simulink model "hcu_main_ADASwEPS"  (Simulink 8.2)
settings: Solver=FixedStepDiscrete  StartTime=0.0  StopTime=inf  FixedStep=0.001  RelTol=1e-3
PostLoadFcn:
  | , if any(exist('dsrtsu_mdlpostloadfcn', 'file') == [2, 3, 6]), try dsrtsu_mdlpostloadfcn('Execute', bdroot); catch fprintf('Error in PostLoadFcn (dsrtsu_mdlpostloadfcn) for model "%s":\n %s\n', bdroot, lasterr); end, end,
values from neighbouring files (symbols this model uses):
  C_TASK_1MS_S = (	C_TICK_TIME_S       )    [hcu_local_hdr.m]    (also in temp_ovrd_values.m = double(	0.001                  ))
  C_TICK_TIME_S = single(	0.005	    	)    [hcu_local_hdr.m]
  ENUM_EPSLFCSTATUS_ACTIVE = uint8(  2  )    [hcu_local_hdr.m]
  ENUM_EPSLFCSTATUS_TRANSITION = uint8(  3  )    [hcu_local_hdr.m]
  ENUM_EPSLKASTATUS_ACTIVE = uint8(  2  )    [hcu_local_hdr.m]
  ENUM_EPSMODEREQ_ANGLE = uint8(  1  )    [hcu_local_hdr.m]
  ENUM_EPSMODEREQ_INTERNAL = uint8(  0  )    [hcu_local_hdr.m]
  ENUM_EPSMODEREQ_TORQUE = uint8(  2  )    [hcu_local_hdr.m]
  ENUM_GEARPOSN_1ST = uint8(  1  )    [hcu_local_hdr.m]
  ENUM_GEARPOSN_2ND = uint8(  2  )    [hcu_local_hdr.m]
  ENUM_GEARPOSN_3RD = uint8(  3  )    [hcu_local_hdr.m]
  ENUM_GEARPOSN_4TH = uint8(  4  )    [hcu_local_hdr.m]
  ENUM_GEARPOSN_5TH = uint8(  5  )    [hcu_local_hdr.m]
  ENUM_GEARPOSN_6TH = uint8(  6  )    [hcu_local_hdr.m]
  ENUM_GEARPOSN_R = uint8(  7  )    [hcu_local_hdr.m]
  FALSE = boolean( 0 )    [hcu_local_hdr.m]
  TRUE = boolean( 1 )    [hcu_local_hdr.m]
undefined symbols (not defined in the file or in its folder): AISP_EPSCurrent_pct, AISP_TqASensorDelta_pct, AISP_TqBSensorDelta_pct, dHAL_IN, hal, INVALID_ABS1_TIMEOUT, INVALID_ABS2_TIMEOUT, INVALID_ABS3_TIMEOUT, INVALID_ABS4_TIMEOUT, INVALID_AC1_TIMEOUT, INVALID_ADASTORQ_REQ, INVALID_BCM1_TIMEOUT, INVALID_BCM2_TIMEOUT, INVALID_BOOSTER_VAC, INVALID_CSW1_TIMEOUT, INVALID_CUR_VEHDECE, INVALID_CURBRAKEDECE_REQ, INVALID_CURSTEERANG_REQ, INVALID_CURSTEERTQ_REQ, INVALID_ECM1_TIMEOUT, INVALID_ECM2_TIMEOUT, INVALID_ECM3_TIMEOUT, INVALID_ECM9_TIMEOUT, INVALID_ENG_TORQUE_FRICTIONAL, INVALID_ENG_TORQUE_INDICATED, INVALID_ENG_TORQUE_INDICATEDCOR, INVALID_ENG_TQ_MAX, INVALID_ENG_TQ_MIN, INVALID_EPAS2_TIMEOUT, INVALID_EPAS3_TIMEOUT, INVALID_EPB1_TIMEOUT, INVALID_EPS_BATTVOLT, INVALID_ESC_BATTVOLT, INVALID_GRADE, INVALID_HCU3_TIMEOUT, INVALID_HCU4_TIMEOUT, INVALID_HMI1_TIMEOUT, INVALID_HMI2_TIMEOUT, INVALID_LAT_ACC, INVALID_LONG_ACC, INVALID_MC_PRESSURE, INVALID_METER1_TIMEOUT, INVALID_METER3_TIMEOUT, INVALID_METER_VEHSPD, INVALID_ODO_METER, INVALID_OUTSIDE_TEMP, INVALID_PARKBRAKEBIND_STAT, INVALID_PEDALTQ_REQ, INVALID_SAS1_TIMEOUT, INVALID_SAS_ANGLE, INVALID_SHIFTER_POSN, INVALID_TCM1_TIMEOUT, INVALID_TCM2_TIMEOUT, INVALID_VCU1_TIMEOUT, INVALID_VCU2_TIMEOUT, INVALID_VEH_CRASH, INVALID_VEH_SPD, INVALID_WHEEL_SPD, INVALID_YAW_RATE, KHAL_MssgIdObj1_num ... (+8)
libraries: simulink x147, hcu_lib x38, rti1401lib_dio_type3 x4, rtimmsu_dsrtlib x3, app x1, rtiethernetudplib x1, rti1401lib_adc_type4 x1, rti1401lib_dac_type3 x1, inp x1, lidr x1, outp x1
(part 13 of 15)

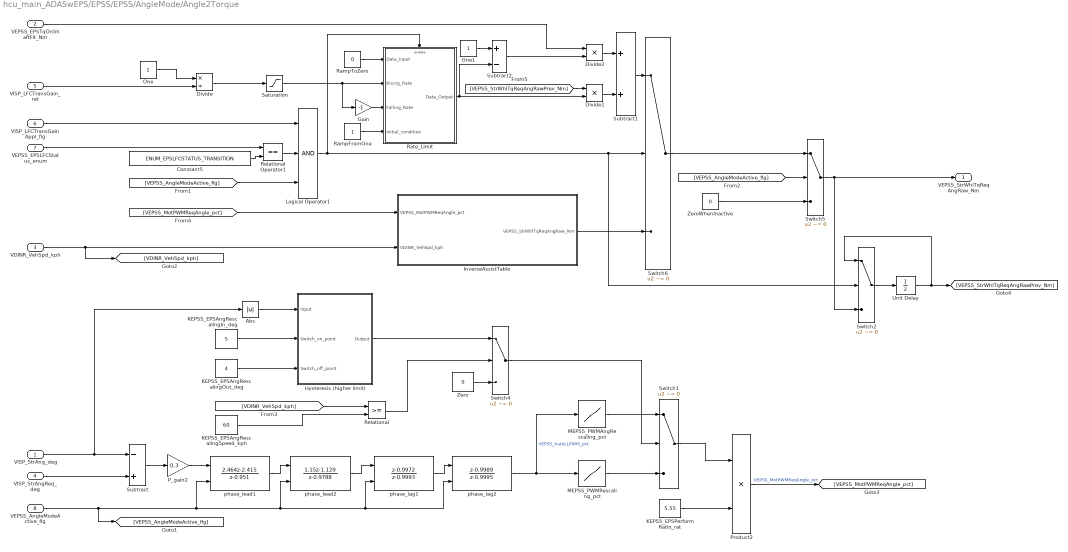
== system hcu_main_ADASwEPS/EPSS/EPSS/AngleMode/Angle2Torque ==
  VISP_StrAng_deg : Inport
  VEPSS_EPSTqOnShaftFlt_Nm : Inport  Port=2
  VDINR_VehSpd_kph : Inport  Port=3
  VISP_StrAngReq_deg : Inport  Port=4
  VISP_LFCTransGain_rat : Inport  Port=5
  VISP_LFCTransGainAppl_flg : Inport  Port=6
  VEPSS_EPSLFCStatus_enum : Inport  Port=7
  VEPSS_AngleModeActive_flg : Inport  Port=8
  Abs : Abs
  Constant5 : Constant  Value=ENUM_EPSLFCSTATUS_TRANSITION
  Divide : Product  Inputs=*/
  Divide1 : Product  Inputs=**
  Divide2 : Product  Inputs=**
  Gain : Gain  Gain=-1
  Hysteresis (higher limit) : Subsystem  TreatAsAtomicUnit=on
  InverseAssistTable : Subsystem
  KEPSS_EPSAngRescalingIn_deg : Constant  Value=5  SampleTime=-1
  KEPSS_EPSAngRescalingOut_deg : Constant  Value=4  SampleTime=-1
  KEPSS_EPSAngRescalingSpeed_kph : Constant  Value=60  SampleTime=-1
  KEPSS_EPSPerformRatio_rat : Constant  Value=5.55  SampleTime=-1
  Logical Operator1 : Logic  Inputs=3  AllPortsSameDT=off  OutDataTypeStr=boolean
  MEPSS_PWMAngRescaling_pct : Lookup  InputValues=[-100 -0.1 0 0.1 100]  Table=[-100 -0.1 0 0.1 100]  LookUpMeth=Interpolation-Use End Values
      settings: AttributesFormatString="Input=\"%<InputValues>\"\\nOutput=\"%<Table>\""
  MEPSS_PWMRescaling_pct : Lookup  InputValues=[-100 -0.1 0 0.1 100]  Table=[-100 -2.2 0 2.6 100]  LookUpMeth=Interpolation-Use End Values
      settings: AttributesFormatString="Input=\"%<InputValues>\"\\nOutput=\"%<Table>\""
  One : Constant
  One1 : Constant
  P_gain2 : Gain  Gain=0.3
  Product2 : Product  RndMeth=Zero
  RampFromOne : Constant
  RampToZero : Constant  Value=0
  Rate_Limit : Subsystem  TreatAsAtomicUnit=on
  "Relational " : RelationalOperator  OutDataTypeStr=boolean
  Relational Operator1 : RelationalOperator  Operator===  OutDataTypeStr=boolean
  Saturation : Saturate  UpperLimit=inf  LowerLimit=0
  Subtract : Sum  Inputs=-+
  Subtract1 : Sum
  Subtract2 : Sum  Inputs=+-
  Switch{1..2,4..6} (5 alike) : Switch  Criteria=u2 ~= 0
  Unit Delay : UnitDelay  SampleTime=-1
  Zero : Constant  Value=0  SampleTime=-1
  ZeroWhenInactive : Constant  Value=0
  phase_lag1 : DiscreteTransferFcn  Numerator=[1 -0.9972]  Denominator=[1 -0.9993]  ExternalReset=Rising
      settings: InputPortMap=u0,r7
  phase_lag2 : DiscreteTransferFcn  Numerator=[1 -0.9989]  Denominator=[1 -0.9995]  ExternalReset=Rising
      settings: InputPortMap=u0,r7
  phase_lead1 : DiscreteTransferFcn  Numerator=[2.464 -2.415]  Denominator=[1 -0.951]  ExternalReset=Rising
      settings: InputPortMap=u0,r7
  phase_lead2 : DiscreteTransferFcn  Numerator=[1.15 -1.129]  Denominator=[1 -0.9788]  ExternalReset=Rising
      settings: InputPortMap=u0,r7
  VEPSS_StrWhlTqReqAngRaw_Nm : Outport
  wires:
  phase_lag2/1 -> MEPSS_PWMRescaling_pct/1, MEPSS_PWMAngRescaling_pct/1  "VEPSS_AutoLLPWM_pct"
  VISP_StrAng_deg/1 -> Subtract/1, Abs/1
  KEPSS_EPSPerformRatio_rat/1 -> Product2/2
  VISP_StrAngReq_deg/1 -> Subtract/2
  MEPSS_PWMRescaling_pct/1 -> Switch1/3
  Product2/1 -> [VEPSS_MotPWMReqAngle_pct]  "VEPSS_MotPWMReqAngle_pct"
  Subtract/1 -> P_gain2/1
  P_gain2/1 -> phase_lead1/1
  phase_lead1/1 -> phase_lead2/1
  phase_lag1/1 -> phase_lag2/1
  phase_lead2/1 -> phase_lag1/1
  MEPSS_PWMAngRescaling_pct/1 -> Switch1/1
  Switch1/1 -> Product2/1
  Switch4/1 -> Switch1/2
  KEPSS_EPSAngRescalingSpeed_kph/1 -> "Relational "/2
  "Relational "/1 -> Switch4/2
  Zero/1 -> Switch4/3
  VEPSS_EPSLFCStatus_enum/1 -> Relational Operator1/1
  Constant5/1 -> Relational Operator1/2
  VISP_LFCTransGainAppl_flg/1 -> Logical Operator1/1
  Relational Operator1/1 -> Logical Operator1/2
  VEPSS_AngleModeActive_flg/1 -> phase_lead2/2, phase_lag2/2, phase_lag1/2, phase_lead1/2, [VEPSS_AngleModeActive_flg]
  InverseAssistTable/1(VEPSS_StrWhlTqReqAngRaw_Nm) -> Switch6/3
  RampToZero/1 -> Rate_Limit/1(Data_Input)
  RampFromOne/1 -> Rate_Limit/4(Initial_condition)
  Logical Operator1/1 -> Switch2/2, Switch6/2, Rate_Limit/Enable
  Divide/1 -> Saturation/1
  Gain/1 -> Rate_Limit/3(Falling_Rate)
  [VEPSS_AngleModeActive_flg] -> Logical Operator1/3
  Switch6/1 -> Switch5/1
  Switch5/1 -> Switch2/3, VEPSS_StrWhlTqReqAngRaw_Nm/1
  [VEPSS_AngleModeActive_flg] -> Switch5/2
  ZeroWhenInactive/1 -> Switch5/3
  VDINR_VehSpd_kph/1 -> [VDINR_VehSpd_kph], InverseAssistTable/2(VDINR_VehSpd_kph)
  [VDINR_VehSpd_kph] -> "Relational "/1
  Abs/1 -> Hysteresis (higher limit)/1(Input)
  KEPSS_EPSAngRescalingIn_deg/1 -> Hysteresis (higher limit)/2(Switch_on_point)
  KEPSS_EPSAngRescalingOut_deg/1 -> Hysteresis (higher limit)/3(Switch_off_point)
  Hysteresis (higher limit)/1(Output) -> Switch4/1
  [VEPSS_MotPWMReqAngle_pct] -> InverseAssistTable/1(VEPSS_MotPWMReqAngle_pct)
  VEPSS_EPSTqOnShaftFlt_Nm/1 -> Divide2/1
  VISP_LFCTransGain_rat/1 -> Divide/2
  One/1 -> Divide/1
  Saturation/1 -> Gain/1, Rate_Limit/2(Rising_Rate)
  Subtract1/1 -> Switch6/1
  Divide1/1 -> Subtract1/2
  Rate_Limit/1(Data_Output) -> Subtract2/2, Divide1/2
  Divide2/1 -> Subtract1/1
  [VEPSS_StrWhlTqReqAngRawPrev_Nm] -> Divide1/1
  Subtract2/1 -> Divide2/2
  One1/1 -> Subtract2/1
  Switch2/1 -> Unit Delay/1
  Unit Delay/1 -> Switch2/1, [VEPSS_StrWhlTqReqAngRawPrev_Nm]

== system hcu_main_ADASwEPS/EPSS/EPSS/EPSMotorPWMRequest/MotorPWMRequestCalculation ==
  VEPSS_EPSMotTqReqRaw_Nm : Inport
  1/KEPSS_PWM2TqGain_rat : Gain
  VEPSS_EPSMotPWMReqRaw_pct : Outport
  wires:
  1/KEPSS_PWM2TqGain_rat/1 -> VEPSS_EPSMotPWMReqRaw_pct/1  "VEPSS_EPSMotPWMReqRaw_pct"
  VEPSS_EPSMotTqReqRaw_Nm/1 -> 1/KEPSS_PWM2TqGain_rat/1

== system hcu_main_ADASwEPS/EPSS/EPSS/EPSMotorPWMRequest/MotorTorqueRequestCalculation ==
  VEPSS_StrWhlTqReqAst_Nm : Inport
  VEPSS_StrWhlTqReqTq_Nm : Inport  Port=2
  VEPSS_StrWhlTqReqAng_Nm : Inport  Port=3
  VEPSS_TorqueModeActive_flg : Inport  Port=4
  VEPSS_AngleModeActive_flg : Inport  Port=5
  VISP_VehSpd_kph : Inport  Port=6
  VISP_LFCTransGain_rat : Inport  Port=7
  VISP_LFCTransGainAppl_flg : Inport  Port=8
  VEPSS_EPSLFCStatus_enum : Inport  Port=9
  VISP_EPSModeReq_enum : Inport  Port=10
  EPSGainDefault : Constant
  KEPSS_PWM2TqGain_rat : Gain
  MEPSS_MotorPWMRescaling_pct : Lookup  InputValues=[-100 -3 0 3 100]  Table=[-250 -3 0 3 250]  LookUpMeth=Interpolation-Use End Values
      settings: AttributesFormatString="Input=\"%<InputValues>\"\\nOutput=\"%<Table>\""
  MEPSS_TqPWMMult_rat : Lookup  InputValues=[-100 -80 -60 -40 -20 -10 0 10 20 40 60 80 100]  Table=[1 1 1 1 1 1 1 1 1 1 1 1 1]  LookUpMeth=Interpolation-Use End Values
      settings: AttributesFormatString="Input=\"%<InputValues>\"\\nOutput=\"%<Table>\""
  MEPSS_TqPWM_pct : Lookup  InputValues=[-10:0.5:10]  Table="[-100\t-95\t-90\t-85\t-80\t-75\t-70\t-65\t-60\t-55\t-50\t-45\t-40\t-35\t-30\t-25\t-20\t-15\t-10\t-5\t0\t5\t10\t15\t20\t25\t30\t35\t40\t45\t50\t55\t60\t65\t70\t75\t80\t85\t90\t95\t100]"  LookUpMeth=Interpolation-Use End Values
      settings: AttributesFormatString="Input=\"%<InputValues>\"\\nOutput=\"%<Table>\""
  Product1 : Product  Inputs=3
  Switch : Switch  Criteria=u2 ~= 0
  Switch1 : Switch  Criteria=u2 ~= 0
  Terminator{,1..3} (4 alike) : Terminator
  VEPSS_EPSMotTqReq_Nm : Outport
  wires:
  MEPSS_TqPWMMult_rat/1 -> Product1/2
  MEPSS_TqPWM_pct/1 -> Product1/1
  VISP_VehSpd_kph/1 -> MEPSS_TqPWMMult_rat/1
  Product1/1 -> MEPSS_MotorPWMRescaling_pct/1
  VEPSS_AngleModeActive_flg/1 -> Switch/2
  VEPSS_StrWhlTqReqAng_Nm/1 -> Switch/1
  Switch1/1 -> Switch/3
  VEPSS_TorqueModeActive_flg/1 -> Switch1/2
  VEPSS_StrWhlTqReqTq_Nm/1 -> Switch1/1
  VEPSS_StrWhlTqReqAst_Nm/1 -> Switch1/3
  Switch/1 -> MEPSS_TqPWM_pct/1
  EPSGainDefault/1 -> Product1/3  "VEPSS_MotTqGain_rat"
  MEPSS_MotorPWMRescaling_pct/1 -> KEPSS_PWM2TqGain_rat/1
  KEPSS_PWM2TqGain_rat/1 -> VEPSS_EPSMotTqReq_Nm/1  "VEPSS_EPSMotTqReq_Nm"
  VISP_LFCTransGain_rat/1 -> Terminator/1
  VISP_LFCTransGainAppl_flg/1 -> Terminator1/1
  VEPSS_EPSLFCStatus_enum/1 -> Terminator2/1
  VISP_EPSModeReq_enum/1 -> Terminator3/1

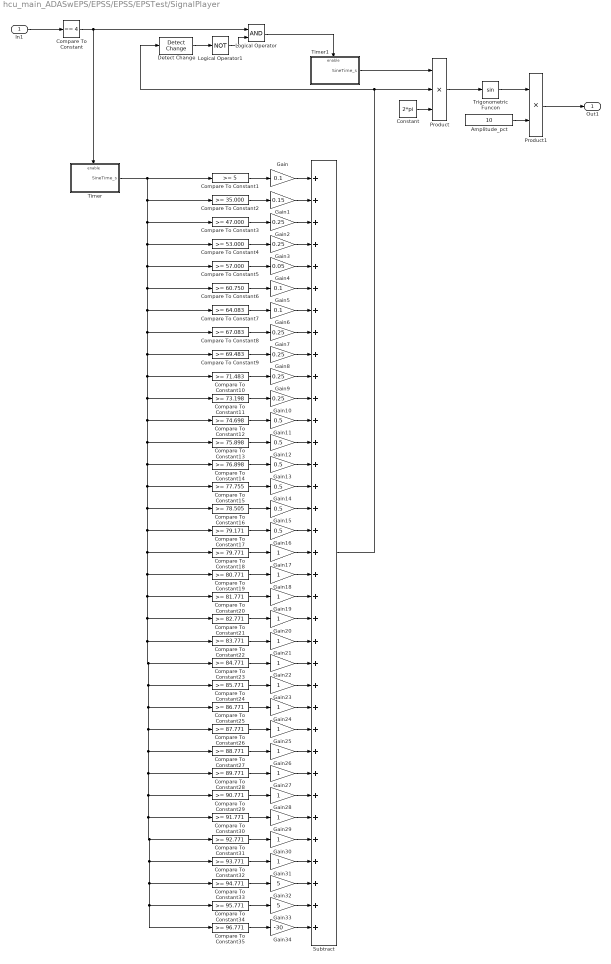
== system hcu_main_ADASwEPS/EPSS/EPSS/EPSTest/SignalPlayer ==
  In1 : Inport
  Amplitude_pct : Constant  Value=10
  Compare To Constant : simulink/Logic and Bit Operations/Compare To Constant  relop===  const=4  OutDataTypeStr=boolean
  Compare To Constant1 : simulink/Logic and Bit Operations/Compare To Constant  relop=>=  const=5  OutDataTypeStr=boolean
  Compare To Constant10 : simulink/Logic and Bit Operations/Compare To Constant  relop=>=  const=71.483  OutDataTypeStr=boolean
  Compare To Constant11 : simulink/Logic and Bit Operations/Compare To Constant  relop=>=  const=73.198  OutDataTypeStr=boolean
  Compare To Constant12 : simulink/Logic and Bit Operations/Compare To Constant  relop=>=  const=74.698  OutDataTypeStr=boolean
  Compare To Constant13 : simulink/Logic and Bit Operations/Compare To Constant  relop=>=  const=75.898  OutDataTypeStr=boolean
  Compare To Constant14 : simulink/Logic and Bit Operations/Compare To Constant  relop=>=  const=76.898  OutDataTypeStr=boolean
  Compare To Constant15 : simulink/Logic and Bit Operations/Compare To Constant  relop=>=  const=77.755  OutDataTypeStr=boolean
  Compare To Constant16 : simulink/Logic and Bit Operations/Compare To Constant  relop=>=  const=78.505  OutDataTypeStr=boolean
  Compare To Constant17 : simulink/Logic and Bit Operations/Compare To Constant  relop=>=  const=79.171  OutDataTypeStr=boolean
  Compare To Constant18 : simulink/Logic and Bit Operations/Compare To Constant  relop=>=  const=79.771  OutDataTypeStr=boolean
  Compare To Constant19 : simulink/Logic and Bit Operations/Compare To Constant  relop=>=  const=80.771  OutDataTypeStr=boolean
  Compare To Constant2 : simulink/Logic and Bit Operations/Compare To Constant  relop=>=  const=35.000  OutDataTypeStr=boolean
  Compare To Constant20 : simulink/Logic and Bit Operations/Compare To Constant  relop=>=  const=81.771  OutDataTypeStr=boolean
  Compare To Constant21 : simulink/Logic and Bit Operations/Compare To Constant  relop=>=  const=82.771  OutDataTypeStr=boolean
  Compare To Constant22 : simulink/Logic and Bit Operations/Compare To Constant  relop=>=  const=83.771  OutDataTypeStr=boolean
  Compare To Constant23 : simulink/Logic and Bit Operations/Compare To Constant  relop=>=  const=84.771  OutDataTypeStr=boolean
  Compare To Constant24 : simulink/Logic and Bit Operations/Compare To Constant  relop=>=  const=85.771  OutDataTypeStr=boolean
  Compare To Constant25 : simulink/Logic and Bit Operations/Compare To Constant  relop=>=  const=86.771  OutDataTypeStr=boolean
  Compare To Constant26 : simulink/Logic and Bit Operations/Compare To Constant  relop=>=  const=87.771  OutDataTypeStr=boolean
  Compare To Constant27 : simulink/Logic and Bit Operations/Compare To Constant  relop=>=  const=88.771  OutDataTypeStr=boolean
  Compare To Constant28 : simulink/Logic and Bit Operations/Compare To Constant  relop=>=  const=89.771  OutDataTypeStr=boolean
  Compare To Constant29 : simulink/Logic and Bit Operations/Compare To Constant  relop=>=  const=90.771  OutDataTypeStr=boolean
  Compare To Constant3 : simulink/Logic and Bit Operations/Compare To Constant  relop=>=  const=47.000  OutDataTypeStr=boolean
  Compare To Constant30 : simulink/Logic and Bit Operations/Compare To Constant  relop=>=  const=91.771  OutDataTypeStr=boolean
  Compare To Constant31 : simulink/Logic and Bit Operations/Compare To Constant  relop=>=  const=92.771  OutDataTypeStr=boolean
  Compare To Constant32 : simulink/Logic and Bit Operations/Compare To Constant  relop=>=  const=93.771  OutDataTypeStr=boolean
  Compare To Constant33 : simulink/Logic and Bit Operations/Compare To Constant  relop=>=  const=94.771  OutDataTypeStr=boolean
  Compare To Constant34 : simulink/Logic and Bit Operations/Compare To Constant  relop=>=  const=95.771  OutDataTypeStr=boolean
  Compare To Constant35 : simulink/Logic and Bit Operations/Compare To Constant  relop=>=  const=96.771  OutDataTypeStr=boolean
  Compare To Constant4 : simulink/Logic and Bit Operations/Compare To Constant  relop=>=  const=53.000  OutDataTypeStr=boolean
  Compare To Constant5 : simulink/Logic and Bit Operations/Compare To Constant  relop=>=  const=57.000  OutDataTypeStr=boolean
  Compare To Constant6 : simulink/Logic and Bit Operations/Compare To Constant  relop=>=  const=60.750  OutDataTypeStr=boolean
  Compare To Constant7 : simulink/Logic and Bit Operations/Compare To Constant  relop=>=  const=64.083  OutDataTypeStr=boolean
  Compare To Constant8 : simulink/Logic and Bit Operations/Compare To Constant  relop=>=  const=67.083  OutDataTypeStr=boolean
  Compare To Constant9 : simulink/Logic and Bit Operations/Compare To Constant  relop=>=  const=69.483  OutDataTypeStr=boolean
  Constant : Constant  Value=2*pi  OutDataTypeStr=single
  Detect Change : simulink/Logic and Bit Operations/Detect Change  vinit=0  InputProcessing=Inherited  OutDataTypeStr=boolean
  Gain : Gain  Gain=0.1
  Gain1 : Gain  Gain=0.15
  Gain{2..3,7..10} (6 alike) : Gain  Gain=0.25
  Gain{11..16} (6 alike) : Gain  Gain=0.5
  Gain{17..31} (15 alike) : Gain
  Gain32 : Gain  Gain=5
  Gain33 : Gain  Gain=5
  Gain34 : Gain  Gain=-30
  Gain4 : Gain  Gain=0.05
  Gain5 : Gain  Gain=0.1
  Gain6 : Gain  Gain=0.1
  Logical Operator : Logic  AllPortsSameDT=off  OutDataTypeStr=boolean
  Logical Operator1 : Logic  Operator=NOT  AllPortsSameDT=off  OutDataTypeStr=boolean
  Product : Product  Inputs=3  RndMeth=Zero
  Product1 : Product  RndMeth=Zero
  Subtract : Sum  Inputs=35
  Timer : Subsystem
  Timer1 : Subsystem
  Trigonometric Funcon : Trigonometry
  Out1 : Outport
  wires:
  Subtract/1 -> Product/2, Detect Change/1
  Product/1 -> Trigonometric Funcon/1
  Amplitude_pct/1 -> Product1/2
  Trigonometric Funcon/1 -> Product1/1
  Constant/1 -> Product/3
  Compare To Constant/1 -> Logical Operator/1, Timer/Enable
  In1/1 -> Compare To Constant/1
  Timer/1(SineTime_s) -> Compare To Constant2/1, Compare To Constant8/1, Compare To Constant35/1, Compare To Constant34/1, Compare To Constant33/1, Compare To Constant32/1, Compare To Constant31/1, Compare To Constant30/1, Compare To Constant29/1, Compare To Constant28/1, Compare To Constant27/1, Compare To Constant26/1, Compare To Constant25/1, Compare To Constant24/1, Compare To Constant23/1, Compare To Constant22/1, Compare To Constant21/1, Compare To Constant20/1, Compare To Constant19/1, Compare To Constant18/1, Compare To Constant17/1, Compare To Constant16/1, Compare To Constant15/1, Compare To Constant14/1, Compare To Constant13/1, Compare To Constant12/1, Compare To Constant11/1, Compare To Constant10/1, Compare To Constant9/1, Compare To Constant7/1, Compare To Constant6/1, Compare To Constant5/1, Compare To Constant4/1, Compare To Constant3/1, Compare To Constant1/1
  Compare To Constant1/1 -> Gain/1
  Gain/1 -> Subtract/1
  Compare To Constant2/1 -> Gain1/1
  Gain1/1 -> Subtract/2
  Compare To Constant3/1 -> Gain2/1
  Gain2/1 -> Subtract/3
  Compare To Constant4/1 -> Gain3/1
  Gain3/1 -> Subtract/4
  Compare To Constant5/1 -> Gain4/1
  Gain4/1 -> Subtract/5
  Compare To Constant6/1 -> Gain5/1
  Gain5/1 -> Subtract/6
  Compare To Constant7/1 -> Gain6/1
  Gain6/1 -> Subtract/7
  Compare To Constant8/1 -> Gain7/1
  Gain7/1 -> Subtract/8
  Compare To Constant9/1 -> Gain8/1
  Gain8/1 -> Subtract/9
  Compare To Constant10/1 -> Gain9/1
  Gain9/1 -> Subtract/10
  Compare To Constant11/1 -> Gain10/1
  Gain10/1 -> Subtract/11
  Compare To Constant12/1 -> Gain11/1
  Gain11/1 -> Subtract/12
  Compare To Constant13/1 -> Gain12/1
  Gain12/1 -> Subtract/13
  Compare To Constant14/1 -> Gain13/1
  Gain13/1 -> Subtract/14
  Compare To Constant15/1 -> Gain14/1
  Gain14/1 -> Subtract/15
  Compare To Constant16/1 -> Gain15/1
  Gain15/1 -> Subtract/16
  Compare To Constant17/1 -> Gain16/1
  Gain16/1 -> Subtract/17
  Compare To Constant18/1 -> Gain17/1
  Gain17/1 -> Subtract/18
  Compare To Constant19/1 -> Gain18/1
  Gain18/1 -> Subtract/19
  Compare To Constant20/1 -> Gain19/1
  Gain19/1 -> Subtract/20
  Compare To Constant21/1 -> Gain20/1
  Gain20/1 -> Subtract/21
  Compare To Constant22/1 -> Gain21/1
  Gain21/1 -> Subtract/22
  Compare To Constant23/1 -> Gain22/1
  Gain22/1 -> Subtract/23
  Compare To Constant24/1 -> Gain23/1
  Gain23/1 -> Subtract/24
  Compare To Constant25/1 -> Gain24/1
  Gain24/1 -> Subtract/25
  Compare To Constant26/1 -> Gain25/1
  Gain25/1 -> Subtract/26
  Compare To Constant27/1 -> Gain26/1
  Gain26/1 -> Subtract/27
  Compare To Constant28/1 -> Gain27/1
  Gain27/1 -> Subtract/28
  Compare To Constant29/1 -> Gain28/1
  Gain28/1 -> Subtract/29
  Compare To Constant30/1 -> Gain29/1
  Gain29/1 -> Subtract/30
  Compare To Constant31/1 -> Gain30/1
  Gain30/1 -> Subtract/31
  Compare To Constant32/1 -> Gain31/1
  Gain31/1 -> Subtract/32
  Compare To Constant33/1 -> Gain32/1
  Gain32/1 -> Subtract/33
  Compare To Constant34/1 -> Gain33/1
  Gain33/1 -> Subtract/34
  Compare To Constant35/1 -> Gain34/1
  Gain34/1 -> Subtract/35
  Product1/1 -> Out1/1
  Timer1/1(SineTime_s) -> Product/1
  Logical Operator/1 -> Timer1/Enable
  Detect Change/1 -> Logical Operator1/1
  Logical Operator1/1 -> Logical Operator/2

== system hcu_main_ADASwEPS/EPSS/EPSS/EPSTest/Timer ==
  Enable : EnablePort  StatesWhenEnabling=reset
  C_TASK_1MS_S : Constant  Value=C_TASK_1MS_S
  Sum : Sum  Inputs=|++
  Unit Delay : UnitDelay  SampleTime=-1
  Unit Delay1 : UnitDelay  SampleTime=-1
  SineTime_s : Outport  OutputWhenDisabled=reset  InitialOutput=[0]
  wires:
  Unit Delay1/1 -> Sum/1
  Unit Delay/1 -> Sum/2
  Sum/1 -> SineTime_s/1, Unit Delay/1  "SineTime_s"
  C_TASK_1MS_S/1 -> Unit Delay1/1

== system hcu_main_ADASwEPS/ISP/PassThrough/EPSDegTest/Timer ==
  Enable : EnablePort  StatesWhenEnabling=reset
  C_TASK_1MS_S : Constant  Value=C_TASK_1MS_S
  Sum : Sum  Inputs=|++
  Unit Delay : UnitDelay  SampleTime=-1
  Unit Delay1 : UnitDelay  SampleTime=-1
  SineTime_s : Outport  OutputWhenDisabled=reset  InitialOutput=[0]
  wires:
  Unit Delay1/1 -> Sum/1
  Unit Delay/1 -> Sum/2
  Sum/1 -> SineTime_s/1, Unit Delay/1  "SineTime_s"
  C_TASK_1MS_S/1 -> Unit Delay1/1

== system hcu_main_ADASwEPS/ISP/TqProcessing/TqSensorAZero/Latch ==
  in : Inport
  update : Inport  Port=2
  Delay : Delay  DelayLength=1  InitialCondition=50
  Switch2 : Switch  Criteria=u2 ~= 0  Threshold=0.5
      settings: AttributesFormatString=<Criteria=%<Criteria>>
  out : Outport
  wires:
  Delay/1 -> Switch2/3
  in/1 -> Switch2/1
  Switch2/1 -> out/1, Delay/1
  update/1 -> Switch2/2

== system hcu_main_ADASwEPS/ISP/TqProcessing/TqSensorAZero/Timer ==
  Enable : EnablePort  StatesWhenEnabling=reset
  C_TASK_1MS_S : Constant  Value=C_TASK_1MS_S
  Sum : Sum  Inputs=|++
  Unit Delay : UnitDelay  SampleTime=-1
  Unit Delay1 : UnitDelay  SampleTime=-1
  Time_s : Outport  OutputWhenDisabled=reset  InitialOutput=[0]
  wires:
  Unit Delay1/1 -> Sum/1
  Unit Delay/1 -> Sum/2
  Sum/1 -> Time_s/1, Unit Delay/1  "Time_s"
  C_TASK_1MS_S/1 -> Unit Delay1/1

== system hcu_main_ADASwEPS/ISP/TqProcessing/TqSensorBZero/Latch ==
  in : Inport
  update : Inport  Port=2
  Delay : Delay  DelayLength=1  InitialCondition=50
  Switch2 : Switch  Criteria=u2 ~= 0  Threshold=0.5
      settings: AttributesFormatString=<Criteria=%<Criteria>>
  out : Outport
  wires:
  update/1 -> Switch2/2
  Switch2/1 -> Delay/1, out/1
  in/1 -> Switch2/1
  Delay/1 -> Switch2/3

== system hcu_main_ADASwEPS/ISP/TqProcessing/TqSensorBZero/Timer ==
  Enable : EnablePort  StatesWhenEnabling=reset
  C_TASK_1MS_S : Constant  Value=C_TASK_1MS_S
  Sum : Sum  Inputs=|++
  Unit Delay : UnitDelay  SampleTime=-1
  Unit Delay1 : UnitDelay  SampleTime=-1
  Time_s : Outport  OutputWhenDisabled=reset  InitialOutput=[0]
  wires:
  C_TASK_1MS_S/1 -> Unit Delay1/1
  Sum/1 -> Unit Delay/1, Time_s/1  "Time_s"
  Unit Delay/1 -> Sum/2
  Unit Delay1/1 -> Sum/1

== system hcu_main_ADASwEPS/OSP/OSP/CheckSum Calculation/Byte0 ==
  BISP_outputs : Inport
  Bus Selector : BusSelector  OutputSignals=VISP_StrAng_deg
  Data Type Conversion : DataTypeConversion  OutDataTypeStr=uint16
  Data Type Conversion1 : DataTypeConversion  OutDataTypeStr=uint16
  Data Type Conversion2 : DataTypeConversion  OutDataTypeStr=uint8
  Data Type Conversion3 : DataTypeConversion  OutDataTypeStr=uint8
  Extract Bits : simulink/Logic and Bit Operations/Extract Bits  bitsToExtract=Upper half  numBits=8  bitIdxRange=[0 7]  outScalingMode=Preserve fixed-point scaling
  Extract Bits1 : simulink/Logic and Bit Operations/Extract Bits  bitsToExtract=Lower half  numBits=8  bitIdxRange=[0 7]  outScalingMode=Preserve fixed-point scaling
  SAS_Angle_cvt : Subsystem  mask(ConvertOut){gain=0.1, offset=-900}
      mask help:
      | Conversion Formula
      |
      | The conversion formula is
      |
      | raw_value = (physical_value - Offset) / Factor
      |
      | where physical_value is the value of the signal after it is saturated using the specified Min and Max values. raw_value is the packed signal value.
  Shift Arithmetic : ArithShift  BitShiftNumber=8
  Byte0 : Outport
  ForByte1 : Outport  Port=2
  wires:
  BISP_outputs/1 -> Bus Selector/1
  Bus Selector/1 -> SAS_Angle_cvt/1(value)  "<VISP_StrAng_deg>"
  SAS_Angle_cvt/1(raw32) -> Data Type Conversion/1
  Data Type Conversion2/1 -> ForByte1/1
  Data Type Conversion1/1 -> Shift Arithmetic/1
  Extract Bits/1 -> Data Type Conversion1/1
  Shift Arithmetic/1 -> Data Type Conversion3/1
  Data Type Conversion3/1 -> Byte0/1
  Extract Bits1/1 -> Data Type Conversion2/1
  Data Type Conversion/1 -> Extract Bits/1, Extract Bits1/1

== system hcu_main_ADASwEPS/OSP/OSP/CheckSum Calculation/Byte1 ==
  ForByte1 : Inport
  Data Type Conversion3 : DataTypeConversion  OutDataTypeStr=uint8
  Byte1 : Outport
  wires:
  Data Type Conversion3/1 -> Byte1/1
  ForByte1/1 -> Data Type Conversion3/1

== system hcu_main_ADASwEPS/OSP/OSP/CheckSum Calculation/Byte2 ==
  Constant1 : Constant  Value=0
  Data Type Conversion3 : DataTypeConversion  OutDataTypeStr=uint8
  Byte2 : Outport
  wires:
  Constant1/1 -> Data Type Conversion3/1
  Data Type Conversion3/1 -> Byte2/1

== system hcu_main_ADASwEPS/OSP/OSP/CheckSum Calculation/Byte3 ==
  BISP_outputs : Inport
  Bus Selector : BusSelector  OutputSignals=VISP_StrAngSensorValid_flg,VISP_StrAngValid_flg
  Data Type Conversion1 : DataTypeConversion  OutDataTypeStr=uint8
  Data Type Conversion2 : DataTypeConversion  OutDataTypeStr=uint8
  Data Type Conversion3 : DataTypeConversion  OutDataTypeStr=uint8
  Sum : Sum  Inputs=2
  bit1 : ArithShift  BitShiftNumber=-1
  Byte3 : Outport
  wires:
  Sum/1 -> Data Type Conversion3/1
  BISP_outputs/1 -> Bus Selector/1
  bit1/1 -> Sum/2
  Data Type Conversion3/1 -> Byte3/1
  Data Type Conversion1/1 -> Sum/1
  Data Type Conversion2/1 -> bit1/1
  Bus Selector/1 -> Data Type Conversion1/1  "<VISP_StrAngSensorValid_flg>"
  Bus Selector/2 -> Data Type Conversion2/1  "<VISP_StrAngValid_flg>"

== system hcu_main_ADASwEPS/OSP/OSP/CheckSum Calculation/ChecksumCalculation ==
  Byte0 : Inport
  Byte1 : Inport  Port=2
  Byte2 : Inport  Port=3
  Byte3 : Inport  Port=4
  SAS_MsgCount : Inport  Port=5
  Bitwise Operator1 : simulink/Logic and Bit Operations/Bitwise Operator  logicop=XOR  UseBitMask=off  NumInputPorts=4  BitMask=bin2dec('11011001')  BitMaskRealWorld=Stored Integer
  Bitwise Operator2 : simulink/Logic and Bit Operations/Bitwise Operator  logicop=XOR  UseBitMask=off  NumInputPorts=3  BitMask=bin2dec('11011001')  BitMaskRealWorld=Stored Integer
  Data Type Conversion{1,3,6..9} (6 alike) : DataTypeConversion  OutDataTypeStr=uint8
  Extract Bits5 : simulink/Logic and Bit Operations/Extract Bits  bitsToExtract=Lower half  numBits=8  bitIdxRange=[0 7]  outScalingMode=Preserve fixed-point scaling
  Extract Bits6 : simulink/Logic and Bit Operations/Extract Bits  bitsToExtract=Upper half  numBits=8  bitIdxRange=[0 7]  outScalingMode=Preserve fixed-point scaling
  Shift Arithmetic2 : ArithShift  BitShiftNumber=4
  Message_Checksum : Outport
  wires:
  Byte1/1 -> Data Type Conversion3/1
  Extract Bits6/1 -> Data Type Conversion7/1
  Extract Bits5/1 -> Data Type Conversion8/1
  Data Type Conversion7/1 -> Shift Arithmetic2/1
  Byte2/1 -> Data Type Conversion6/1
  Byte3/1 -> Data Type Conversion9/1
  Byte0/1 -> Data Type Conversion1/1
  Data Type Conversion1/1 -> Bitwise Operator1/1
  Data Type Conversion3/1 -> Bitwise Operator1/2
  Data Type Conversion6/1 -> Bitwise Operator1/3
  Data Type Conversion9/1 -> Bitwise Operator1/4
  Bitwise Operator1/1 -> Extract Bits6/1, Extract Bits5/1
  Shift Arithmetic2/1 -> Bitwise Operator2/1
  Data Type Conversion8/1 -> Bitwise Operator2/2
  SAS_MsgCount/1 -> Bitwise Operator2/3
  Bitwise Operator2/1 -> Message_Checksum/1

== system hcu_main_ADASwEPS/OSP/OSP/CheckSum Calculation1/Byte0 ==
  Data Type Conversion3 : DataTypeConversion  OutDataTypeStr=uint8
  Elect_PWR_Consumpt : Constant  Value=0
  Elect_PWR_Consumpt_cvt : Subsystem  mask(ConvertOut){gain=0.5, offset=0}
      mask help:
      | Conversion Formula
      |
      | The conversion formula is
      |
      | raw_value = (physical_value - Offset) / Factor
      |
      | where physical_value is the value of the signal after it is saturated using the specified Min and Max values. raw_value is the packed signal value.
  Byte0 : Outport
  wires:
  Elect_PWR_Consumpt/1 -> Elect_PWR_Consumpt_cvt/1(value)
  Data Type Conversion3/1 -> Byte0/1
  Elect_PWR_Consumpt_cvt/1(raw32) -> Data Type Conversion3/1

== system hcu_main_ADASwEPS/OSP/OSP/CheckSum Calculation1/Byte1 ==
  BISP_outputs : Inport
  Bus Selector : BusSelector  OutputSignals=VISP_EPSTqOnShaftValid_flg,VISP_StrAngValid_flg
  Constant : Constant  Value=TRUE
  Data Type Conversion{1..4} (4 alike) : DataTypeConversion  OutDataTypeStr=uint8
  EpasFailed : Constant  Value=FALSE
  Logical Operator : Logic  Operator=NOT  AllPortsSameDT=off  OutDataTypeStr=boolean
  Sum : Sum  Inputs=3
  Terminator : Terminator
  bit6 : ArithShift  BitShiftNumber=-6
  bit7 : ArithShift  BitShiftNumber=-7
  Byte1 : Outport
  wires:
  Sum/1 -> Data Type Conversion3/1
  BISP_outputs/1 -> Bus Selector/1
  bit6/1 -> Sum/2
  Data Type Conversion3/1 -> Byte1/1
  Data Type Conversion1/1 -> Sum/1
  Data Type Conversion2/1 -> bit6/1
  Bus Selector/1 -> Logical Operator/1  "<VISP_EPSTqOnShaftValid_flg>"
  Logical Operator/1 -> Data Type Conversion1/1
  Data Type Conversion4/1 -> bit7/1
  EpasFailed/1 -> Data Type Conversion4/1
  bit7/1 -> Sum/3
  Constant/1 -> Data Type Conversion2/1
  Bus Selector/2 -> Terminator/1  "<VISP_StrAngValid_flg>"

== system hcu_main_ADASwEPS/OSP/OSP/CheckSum Calculation1/Byte2 ==
  BEPSS_outputs : Inport
  Bus Selector : BusSelector  OutputSignals=VEPSS_EPSTqOnShaftFlt_Nm
  Data Type Conversion3 : DataTypeConversion  OutDataTypeStr=uint8
  Steering_Torque_cvt : Subsystem  mask(ConvertOut){gain=0.1794, offset=-22.78}
      mask help:
      | Conversion Formula
      |
      | The conversion formula is
      |
      | raw_value = (physical_value - Offset) / Factor
      |
      | where physical_value is the value of the signal after it is saturated using the specified Min and Max values. raw_value is the packed signal value.
  Byte2 : Outport
  wires:
  Steering_Torque_cvt/1(raw32) -> Data Type Conversion3/1
  Data Type Conversion3/1 -> Byte2/1
  Bus Selector/1 -> Steering_Torque_cvt/1(value)  "<VEPSS_EPSTqOnShaftFlt_Nm>"
  BEPSS_outputs/1 -> Bus Selector/1

== system hcu_main_ADASwEPS/OSP/OSP/CheckSum Calculation1/Byte3 ==
  BISP_outputs : Inport
  Bus Selector : BusSelector  OutputSignals=VISP_RelStrAng_deg
  Data Type Conversion : DataTypeConversion  OutDataTypeStr=uint16
  Data Type Conversion1 : DataTypeConversion  OutDataTypeStr=uint16
  Data Type Conversion2 : DataTypeConversion  OutDataTypeStr=uint8
  Data Type Conversion3 : DataTypeConversion  OutDataTypeStr=uint8
  Extract Bits : simulink/Logic and Bit Operations/Extract Bits  bitsToExtract=Upper half  numBits=8  bitIdxRange=[0 7]  outScalingMode=Preserve fixed-point scaling
  Extract Bits1 : simulink/Logic and Bit Operations/Extract Bits  bitsToExtract=Lower half  numBits=8  bitIdxRange=[0 7]  outScalingMode=Preserve fixed-point scaling
  R_SAS_Angle_cvt : Subsystem  mask(ConvertOut){gain=0.1, offset=-1400}
      mask help:
      | Conversion Formula
      |
      | The conversion formula is
      |
      | raw_value = (physical_value - Offset) / Factor
      |
      | where physical_value is the value of the signal after it is saturated using the specified Min and Max values. raw_value is the packed signal value.
  Shift Arithmetic : ArithShift  BitShiftNumber=8
  Byte3 : Outport
  ForByte4 : Outport  Port=2
  wires:
  BISP_outputs/1 -> Bus Selector/1
  Bus Selector/1 -> R_SAS_Angle_cvt/1(value)  "<VISP_RelStrAng_deg>"
  R_SAS_Angle_cvt/1(raw32) -> Data Type Conversion/1
  Data Type Conversion2/1 -> ForByte4/1
  Data Type Conversion1/1 -> Shift Arithmetic/1
  Extract Bits/1 -> Data Type Conversion1/1
  Shift Arithmetic/1 -> Data Type Conversion3/1
  Data Type Conversion3/1 -> Byte3/1
  Extract Bits1/1 -> Data Type Conversion2/1
  Data Type Conversion/1 -> Extract Bits/1, Extract Bits1/1

== system hcu_main_ADASwEPS/OSP/OSP/CheckSum Calculation1/ChecksumCalculation ==
  Byte0 : Inport
  Byte1 : Inport  Port=2
  Byte2 : Inport  Port=3
  Byte3 : Inport  Port=4
  Byte4 : Inport  Port=5
  EPAS2_MsgCount : Inport  Port=6
  Bitwise Operator1 : simulink/Logic and Bit Operations/Bitwise Operator  logicop=XOR  UseBitMask=off  NumInputPorts=5  BitMask=bin2dec('11011001')  BitMaskRealWorld=Stored Integer
  Bitwise Operator2 : simulink/Logic and Bit Operations/Bitwise Operator  logicop=XOR  UseBitMask=off  NumInputPorts=3  BitMask=bin2dec('11011001')  BitMaskRealWorld=Stored Integer
  Data Type Conversion{1..3,6..9} (7 alike) : DataTypeConversion  OutDataTypeStr=uint8
  Extract Bits5 : simulink/Logic and Bit Operations/Extract Bits  bitsToExtract=Lower half  numBits=8  bitIdxRange=[0 7]  outScalingMode=Preserve fixed-point scaling
  Extract Bits6 : simulink/Logic and Bit Operations/Extract Bits  bitsToExtract=Upper half  numBits=8  bitIdxRange=[0 7]  outScalingMode=Preserve fixed-point scaling
  Shift Arithmetic2 : ArithShift  BitShiftNumber=4
  Message_Checksum : Outport
  wires:
  Bitwise Operator2/1 -> Message_Checksum/1
  EPAS2_MsgCount/1 -> Bitwise Operator2/3
  Data Type Conversion8/1 -> Bitwise Operator2/2
  Shift Arithmetic2/1 -> Bitwise Operator2/1
  Bitwise Operator1/1 -> Extract Bits5/1, Extract Bits6/1
  Data Type Conversion9/1 -> Bitwise Operator1/4
  Data Type Conversion6/1 -> Bitwise Operator1/3
  Data Type Conversion3/1 -> Bitwise Operator1/2
  Data Type Conversion1/1 -> Bitwise Operator1/1
  Byte0/1 -> Data Type Conversion1/1
  Byte3/1 -> Data Type Conversion9/1
  Byte2/1 -> Data Type Conversion6/1
  Data Type Conversion7/1 -> Shift Arithmetic2/1
  Extract Bits5/1 -> Data Type Conversion8/1
  Extract Bits6/1 -> Data Type Conversion7/1
  Byte1/1 -> Data Type Conversion3/1
  Byte4/1 -> Data Type Conversion2/1
  Data Type Conversion2/1 -> Bitwise Operator1/5

== system hcu_main_ADASwEPS/OSP/OSP/CheckSum Calculation2/Byte0 ==
  BEPSS_outputs : Inport
  Bus Selector : BusSelector  OutputSignals=VEPSS_AckStrAngReq_deg
  CurStrAngReq_cvt : Subsystem  mask(ConvertOut){gain=0.1, offset=-720}
      mask help:
      | Conversion Formula
      |
      | The conversion formula is
      |
      | raw_value = (physical_value - Offset) / Factor
      |
      | where physical_value is the value of the signal after it is saturated using the specified Min and Max values. raw_value is the packed signal value.
  Data Type Conversion : DataTypeConversion  OutDataTypeStr=uint16
  Data Type Conversion1 : DataTypeConversion  OutDataTypeStr=uint16
  Data Type Conversion2 : DataTypeConversion  OutDataTypeStr=uint8
  Data Type Conversion3 : DataTypeConversion  OutDataTypeStr=uint8
  Extract Bits : simulink/Logic and Bit Operations/Extract Bits  bitsToExtract=Upper half  numBits=8  bitIdxRange=[0 7]  outScalingMode=Preserve fixed-point scaling
  Extract Bits1 : simulink/Logic and Bit Operations/Extract Bits  bitsToExtract=Lower half  numBits=8  bitIdxRange=[0 7]  outScalingMode=Preserve fixed-point scaling
  Shift Arithmetic : ArithShift  BitShiftNumber=8
  Byte0 : Outport
  ForByte1 : Outport  Port=2
  wires:
  Data Type Conversion/1 -> Extract Bits1/1, Extract Bits/1
  Extract Bits1/1 -> Data Type Conversion2/1
  Data Type Conversion3/1 -> Byte0/1
  Shift Arithmetic/1 -> Data Type Conversion3/1
  Extract Bits/1 -> Data Type Conversion1/1
  Data Type Conversion1/1 -> Shift Arithmetic/1
  Data Type Conversion2/1 -> ForByte1/1
  CurStrAngReq_cvt/1(raw32) -> Data Type Conversion/1
  Bus Selector/1 -> CurStrAngReq_cvt/1(value)  "<VEPSS_AckStrAngReq_deg>"
  BEPSS_outputs/1 -> Bus Selector/1

== system hcu_main_ADASwEPS/OSP/OSP/CheckSum Calculation2/Byte1 ==
  ForByte1 : Inport
  Data Type Conversion3 : DataTypeConversion  OutDataTypeStr=uint8
  Byte1 : Outport
  wires:
  ForByte1/1 -> Data Type Conversion3/1
  Data Type Conversion3/1 -> Byte1/1

== system hcu_main_ADASwEPS/OSP/OSP/CheckSum Calculation2/Byte2 ==
  BEPSS_outputs : Inport
  Bus Selector : BusSelector  OutputSignals=VEPSS_EPSADASAbReason_enum,VEPSS_EPSLKAStatus_enum
  Data Type Conversion1 : DataTypeConversion  OutDataTypeStr=uint8
  Data Type Conversion3 : DataTypeConversion  OutDataTypeStr=uint8
  Data Type Conversion4 : DataTypeConversion  OutDataTypeStr=uint8
  Sum : Sum  Inputs=2
  bit5 : ArithShift  BitShiftNumber=-5
  Byte2 : Outport
  wires:
  Bus Selector/1 -> Data Type Conversion1/1  "<VEPSS_EPSADASAbReason_enum>"
  Data Type Conversion1/1 -> Sum/1
  BEPSS_outputs/1 -> Bus Selector/1
  Sum/1 -> Data Type Conversion3/1
  Data Type Conversion3/1 -> Byte2/1
  Data Type Conversion4/1 -> bit5/1
  Bus Selector/2 -> Data Type Conversion4/1  "<VEPSS_EPSLKAStatus_enum>"
  bit5/1 -> Sum/2

== system hcu_main_ADASwEPS/OSP/OSP/CheckSum Calculation2/Byte3 ==
  Constant1 : Constant  Value=0
  Data Type Conversion3 : DataTypeConversion  OutDataTypeStr=uint8
  Byte3 : Outport
  wires:
  Data Type Conversion3/1 -> Byte3/1
  Constant1/1 -> Data Type Conversion3/1

== system hcu_main_ADASwEPS/OSP/OSP/CheckSum Calculation2/Byte4 ==
  BEPSS_outputs : Inport
  Bus Selector : BusSelector  OutputSignals=VEPSS_AckStrTqReq_Nm
  CurStrTqReq_cvt : Subsystem  mask(ConvertOut){gain=0.1, offset=-10}
      mask help:
      | Conversion Formula
      |
      | The conversion formula is
      |
      | raw_value = (physical_value - Offset) / Factor
      |
      | where physical_value is the value of the signal after it is saturated using the specified Min and Max values. raw_value is the packed signal value.
  Data Type Conversion3 : DataTypeConversion  OutDataTypeStr=uint8
  Byte4 : Outport
  wires:
  BEPSS_outputs/1 -> Bus Selector/1
  Bus Selector/1 -> CurStrTqReq_cvt/1(value)  "<VEPSS_AckStrTqReq_Nm>"
  CurStrTqReq_cvt/1(raw32) -> Data Type Conversion3/1
  Data Type Conversion3/1 -> Byte4/1

== system hcu_main_ADASwEPS/OSP/OSP/CheckSum Calculation2/Byte5 ==
  Data Type Conversion3 : DataTypeConversion  OutDataTypeStr=uint8
  EPSBattVolt : Constant  Value=12
  EPSBattVolt_cvt : Subsystem  mask(ConvertOut){gain=0.1, offset=0}
      mask help:
      | Conversion Formula
      |
      | The conversion formula is
      |
      | raw_value = (physical_value - Offset) / Factor
      |
      | where physical_value is the value of the signal after it is saturated using the specified Min and Max values. raw_value is the packed signal value.
  Byte5 : Outport
  wires:
  Data Type Conversion3/1 -> Byte5/1
  EPSBattVolt_cvt/1(raw32) -> Data Type Conversion3/1
  EPSBattVolt/1 -> EPSBattVolt_cvt/1(value)

== system hcu_main_ADASwEPS/OSP/OSP/CheckSum Calculation2/Byte6 ==
  BEPSS_outputs : Inport
  Bus Selector : BusSelector  OutputSignals=VEPSS_AckStrTqReqAppl_flg,VEPSS_AckStrAngReqAppl_flg,VEPSS_EPSLFCStatus_enum
  Data Type Conversion{2..5} (4 alike) : DataTypeConversion  OutDataTypeStr=uint8
  Sum : Sum  Inputs=3
  bit2 : ArithShift  BitShiftNumber=-2
  bit4 : ArithShift  BitShiftNumber=-4
  bit5 : ArithShift  BitShiftNumber=-5
  Byte6 : Outport
  wires:
  bit4/1 -> Sum/2
  Bus Selector/2 -> Data Type Conversion4/1  "<VEPSS_AckStrAngReqAppl_flg>"
  Data Type Conversion4/1 -> bit4/1
  Data Type Conversion3/1 -> Byte6/1
  Sum/1 -> Data Type Conversion3/1
  BEPSS_outputs/1 -> Bus Selector/1
  bit2/1 -> Sum/1
  Data Type Conversion2/1 -> bit2/1
  Bus Selector/1 -> Data Type Conversion2/1  "<VEPSS_AckStrTqReqAppl_flg>"
  Data Type Conversion5/1 -> bit5/1
  Bus Selector/3 -> Data Type Conversion5/1  "<VEPSS_EPSLFCStatus_enum>"
  bit5/1 -> Sum/3

== system hcu_main_ADASwEPS/OSP/OSP/CheckSum Calculation2/ChecksumCalculation ==
  Byte0 : Inport
  Byte1 : Inport  Port=2
  Byte2 : Inport  Port=3
  Byte3 : Inport  Port=4
  Byte4 : Inport  Port=5
  Byte5 : Inport  Port=6
  Byte6 : Inport  Port=7
  SAS_MsgCount : Inport  Port=8
  Bitwise Operator1 : simulink/Logic and Bit Operations/Bitwise Operator  logicop=XOR  UseBitMask=off  NumInputPorts=7  BitMask=bin2dec('11011001')  BitMaskRealWorld=Stored Integer
  Bitwise Operator2 : simulink/Logic and Bit Operations/Bitwise Operator  logicop=XOR  UseBitMask=off  NumInputPorts=3  BitMask=bin2dec('11011001')  BitMaskRealWorld=Stored Integer
  Data Type Conversion{1..9} (9 alike) : DataTypeConversion  OutDataTypeStr=uint8
  Extract Bits5 : simulink/Logic and Bit Operations/Extract Bits  bitsToExtract=Lower half  numBits=8  bitIdxRange=[0 7]  outScalingMode=Preserve fixed-point scaling
  Extract Bits6 : simulink/Logic and Bit Operations/Extract Bits  bitsToExtract=Upper half  numBits=8  bitIdxRange=[0 7]  outScalingMode=Preserve fixed-point scaling
  Shift Arithmetic2 : ArithShift  BitShiftNumber=4
  Message_Checksum : Outport
  wires:
  Bitwise Operator2/1 -> Message_Checksum/1
  SAS_MsgCount/1 -> Bitwise Operator2/3
  Data Type Conversion8/1 -> Bitwise Operator2/2
  Shift Arithmetic2/1 -> Bitwise Operator2/1
  Bitwise Operator1/1 -> Extract Bits5/1, Extract Bits6/1
  Data Type Conversion9/1 -> Bitwise Operator1/4
  Data Type Conversion6/1 -> Bitwise Operator1/3
  Data Type Conversion3/1 -> Bitwise Operator1/2
  Data Type Conversion1/1 -> Bitwise Operator1/1
  Byte0/1 -> Data Type Conversion1/1
  Byte3/1 -> Data Type Conversion9/1
  Byte2/1 -> Data Type Conversion6/1
  Data Type Conversion7/1 -> Shift Arithmetic2/1
  Extract Bits5/1 -> Data Type Conversion8/1
  Extract Bits6/1 -> Data Type Conversion7/1
  Byte1/1 -> Data Type Conversion3/1
  Data Type Conversion2/1 -> Bitwise Operator1/5
  Byte4/1 -> Data Type Conversion2/1
  Data Type Conversion4/1 -> Bitwise Operator1/6
  Byte5/1 -> Data Type Conversion4/1
  Data Type Conversion5/1 -> Bitwise Operator1/7
  Byte6/1 -> Data Type Conversion5/1

== system hcu_main_ADASwEPS/RTI Data/RTI Data Store/RTI Data Store/RTI Data Store ==
  RTI Data Store : Subsystem  mask(RTI_DATA_STORE){}
      mask help:
      | RTI Data Store Block. This block is used by RTI to store internal model dependent data. Deleting this block will result in data loss.
      |
      | NEVER DELETE, COPY, OR MODIFY THIS BLOCK!
      mask Help:
      | RTI Data Store Block. This block is used by RTI to store internal model dependent data. Deleting this block will result in data loss.
      | 
      | NEVER DELETE, COPY, OR MODIFY THIS BLOCK!
      mask Display: text(0.5, 0.5, ' ', 'HorizontalAlignment', 'center');

== system hcu_main_ADASwEPS/dHAL_IN/HAL_IN_RadObjDecoder/RObjectPackFrame/RObjects_Decoder_v2 ==
  Status : Inport
  ID : Inport  Port=2
  Byte1 : Inport  Port=3
  Byte2 : Inport  Port=4
  Byte3 : Inport  Port=5
  Byte4 : Inport  Port=6
  Byte5 : Inport  Port=7
  Byte6 : Inport  Port=8
  Byte7 : Inport  Port=9
  Byte8 : Inport  Port=10
  R_Objects_in : Inport  Port=11
  CheckIDs : Subsystem
  ParseFrames : Subsystem
  R_Objects_out : Outport  OutDataTypeStr=Bus: R_Objects
  wires:
  Status/1 -> CheckIDs/1(Status)
  ID/1 -> CheckIDs/2(ID)
  R_Objects_in/1 -> CheckIDs/3(R_Objects_in)
  Byte1/1 -> ParseFrames/2(Byte1)
  Byte2/1 -> ParseFrames/3(Byte2)
  Byte3/1 -> ParseFrames/4(Byte3)
  CheckIDs/1(R_Objects_out) -> ParseFrames/1(R_Objects_in)
  ParseFrames/1(R_Objects_out) -> R_Objects_out/1
  CheckIDs/2(ParseFrame) -> [ParseFrame]
  [ParseFrame] -> ParseFrames/Trigger
  Byte4/1 -> ParseFrames/5(Byte4)
  Byte5/1 -> ParseFrames/6(Byte5)
  Byte6/1 -> ParseFrames/7(Byte6)
  Byte7/1 -> ParseFrames/8(Byte7)
  Byte8/1 -> ParseFrames/9(Byte8)

== system hcu_main_ADASwEPS/dHAL_IN/HAL_IN_VCU/BO__1360_VCU1__8_VCU/ChecksumCalculation ==
  CAN1_Rx : Inport
  Add : Sum  Inputs=16
  Bitwise Operator : simulink/Logic and Bit Operations/Bitwise Operator  logicop=XOR  UseBitMask=off  NumInputPorts=2  BitMask=bin2dec('11011001')  BitMaskRealWorld=Stored Integer
  Bus Selector : BusSelector  OutputSignals=VCU1.RAW_Byte_1,VCU1.RAW_Byte_2,VCU1.RAW_Byte_3,VCU1.RAW_Byte_4,VCU1.RAW_Byte_5,VCU1.RAW_Byte_6,VCU1.RAW_Byte_7,VCU1.RAW_Byte_8,VCU1.VCU1_LifeCount
  Constant1 : Constant  Value=hex2dec('10')  OutDataTypeStr=uint8
  Constant2 : Constant  Value=hex2dec('ff')  OutDataTypeStr=uint8
  Data Type Conversion{,1..23} (24 alike) : DataTypeConversion  OutDataTypeStr=uint8
  Extract Bits{1,3,5,7,9,12,14} (7 alike) : simulink/Logic and Bit Operations/Extract Bits  bitsToExtract=Lower half  numBits=8  bitIdxRange=[0 7]  outScalingMode=Preserve fixed-point scaling
  Extract Bits{2,4,6,8,10..11,13,15} (8 alike) : simulink/Logic and Bit Operations/Extract Bits  bitsToExtract=Upper half  numBits=8  bitIdxRange=[0 7]  outScalingMode=Preserve fixed-point scaling
  Math Function : Math  Operator=mod  SaturateOnIntegerOverflow=on
  Shift Arithmetic{,1..7} (8 alike) : ArithShift  BitShiftNumber=4
  Message_Checksum : Outport
  wires:
  Bus Selector/1 -> Data Type Conversion/1  "<RAW_Byte_1>"
  Extract Bits2/1 -> Data Type Conversion1/1
  Extract Bits1/1 -> Data Type Conversion2/1
  Data Type Conversion1/1 -> Shift Arithmetic/1
  Data Type Conversion/1 -> Extract Bits2/1, Extract Bits1/1
  Extract Bits4/1 -> Data Type Conversion4/1
  Extract Bits3/1 -> Data Type Conversion5/1
  Data Type Conversion4/1 -> Shift Arithmetic1/1
  Data Type Conversion3/1 -> Extract Bits3/1, Extract Bits4/1
  Shift Arithmetic/1 -> Add/1
  Data Type Conversion2/1 -> Add/2
  Shift Arithmetic1/1 -> Add/3
  Data Type Conversion5/1 -> Add/4
  Bus Selector/2 -> Data Type Conversion3/1  "<RAW_Byte_2>"
  Extract Bits6/1 -> Data Type Conversion7/1
  Extract Bits5/1 -> Data Type Conversion8/1
  Data Type Conversion7/1 -> Shift Arithmetic2/1
  Data Type Conversion6/1 -> Extract Bits6/1, Extract Bits5/1
  Shift Arithmetic2/1 -> Add/5
  Data Type Conversion8/1 -> Add/6
  Bus Selector/3 -> Data Type Conversion6/1  "<RAW_Byte_3>"
  Extract Bits8/1 -> Data Type Conversion10/1
  Extract Bits7/1 -> Data Type Conversion11/1
  Data Type Conversion10/1 -> Shift Arithmetic3/1
  Data Type Conversion9/1 -> Extract Bits7/1, Extract Bits8/1
  Shift Arithmetic3/1 -> Add/7
  Data Type Conversion11/1 -> Add/8
  Bus Selector/4 -> Data Type Conversion9/1  "<RAW_Byte_4>"
  Extract Bits10/1 -> Data Type Conversion12/1
  Extract Bits9/1 -> Data Type Conversion13/1
  Data Type Conversion12/1 -> Shift Arithmetic4/1
  Data Type Conversion14/1 -> Extract Bits10/1, Extract Bits9/1
  Shift Arithmetic4/1 -> Add/9
  Data Type Conversion13/1 -> Add/10
  Bus Selector/5 -> Data Type Conversion14/1  "<RAW_Byte_5>"
  Extract Bits11/1 -> Data Type Conversion15/1
  Extract Bits12/1 -> Data Type Conversion16/1
  Data Type Conversion15/1 -> Shift Arithmetic5/1
  Data Type Conversion17/1 -> Extract Bits12/1, Extract Bits11/1
  Shift Arithmetic5/1 -> Add/11
  Data Type Conversion16/1 -> Add/12
  Bus Selector/6 -> Data Type Conversion17/1  "<RAW_Byte_6>"
  Extract Bits13/1 -> Data Type Conversion18/1
  Extract Bits14/1 -> Data Type Conversion19/1
  Data Type Conversion18/1 -> Shift Arithmetic6/1
  Data Type Conversion20/1 -> Extract Bits13/1, Extract Bits14/1
  Shift Arithmetic6/1 -> Add/13
  Data Type Conversion19/1 -> Add/14
  Bus Selector/7 -> Data Type Conversion20/1  "<RAW_Byte_7>"
  Extract Bits15/1 -> Data Type Conversion21/1
  Data Type Conversion21/1 -> Shift Arithmetic7/1
  Data Type Conversion23/1 -> Extract Bits15/1
  Shift Arithmetic7/1 -> Add/15
  Bus Selector/8 -> Data Type Conversion23/1  "<RAW_Byte_8>"
  Data Type Conversion22/1 -> Add/16
  Add/1 -> Bitwise Operator/1
  Constant2/1 -> Bitwise Operator/2
  Bitwise Operator/1 -> Math Function/1
  Constant1/1 -> Math Function/2
  Math Function/1 -> Message_Checksum/1
  CAN1_Rx/1 -> Bus Selector/1
  Bus Selector/9 -> Data Type Conversion22/1  "<VCU1_LifeCount>"
